simulink model "evaporator"  (R2021b)
settings: Solver=VariableStepAuto  StartTime=0.0  StopTime=10.0  RelTol=1e-3
settings Model: Creator=Edwar  LastModifiedBy=Edwar

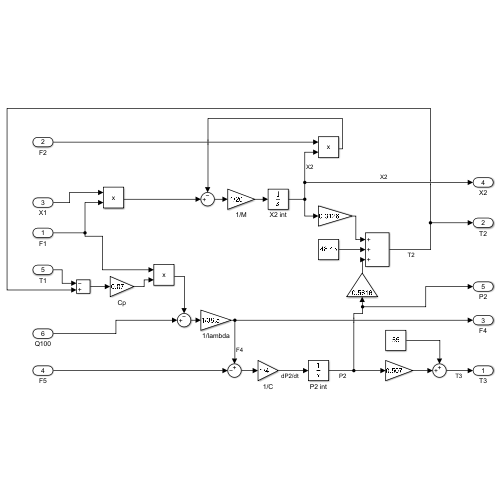
[thumbnail: Simulink's stored preview of the top-level diagram]
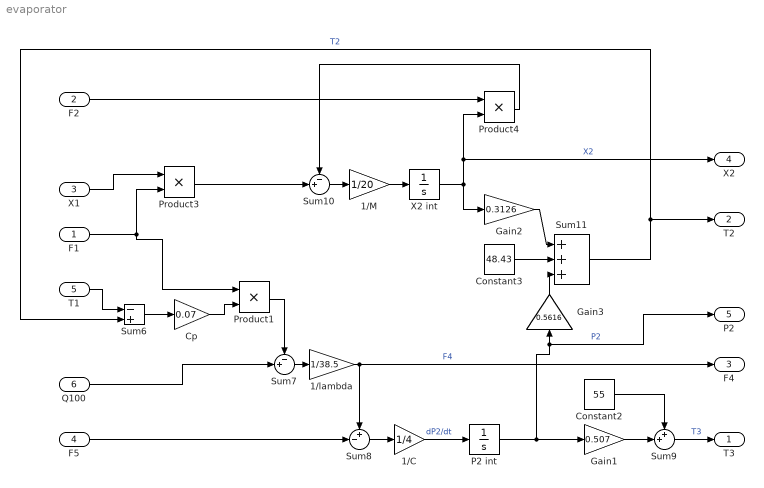
== system evaporator ==
  F1 : Inport
  F2 : Inport  Port=2
  X1 : Inport  Port=3
  F5 : Inport  Port=4
  T1 : Inport  Port=5
  Q100 : Inport  Port=6
  1/C : Gain  Gain=1/4
  1/M : Gain  Gain=1/20
  1/lambda : Gain  Gain=1/38.5
  Constant2 : Constant  Value=55
  Constant3 : Constant  Value=48.43
  Cp : Gain  Gain=0.07
  Gain1 : Gain  Gain=0.507
  Gain2 : Gain  Gain=0.3126
  Gain3 : Gain  Gain=0.5616
  P2 int : Integrator
  Product1 : Product
  Product3 : Product
  Product4 : Product
  Sum10 : Sum  Inputs=-+|
  Sum11 : Sum  Inputs=+++
  Sum6 : Sum  Inputs=-+
  Sum7 : Sum  Inputs=-+|
  Sum8 : Sum  Inputs=+-|
  Sum9 : Sum  Inputs=++|
  X2 int : Integrator
  T3 : Outport
  T2 : Outport  Port=2
  F4 : Outport  Port=3
  X2 : Outport  Port=4
  P2 : Outport  Port=5
  wires:
  P2 int/1 -> P2/1, Gain3/1, Gain1/1  "P2"
  1/lambda/1 -> F4/1, Sum8/1  "F4"
  Sum7/1 -> 1/lambda/1
  Sum6/1 -> Cp/1
  Cp/1 -> Product1/2
  Product1/1 -> Sum7/1
  X1/1 -> Product3/1
  F2/1 -> Product4/1
  Sum10/1 -> 1/M/1
  1/M/1 -> X2 int/1
  Product3/1 -> Sum10/2
  Gain1/1 -> Sum9/2
  X2 int/1 -> X2/1, Product4/2, Gain2/1  "X2"
  F5/1 -> Sum8/2
  F1/1 -> Product1/1, Product3/2
  Sum8/1 -> 1/C/1
  Constant2/1 -> Sum9/1
  Sum11/1 -> T2/1, Sum6/2  "T2"
  Q100/1 -> Sum7/2
  Constant3/1 -> Sum11/2
  T1/1 -> Sum6/1
  Product4/1 -> Sum10/1
  Gain3/1 -> Sum11/3
  1/C/1 -> P2 int/1  "dP2/dt"
  Gain2/1 -> Sum11/1
  Sum9/1 -> T3/1  "T3"
